simulink model "stateSpaceModel"  (R2025a)
settings: Solver=VariableStepAuto  StartTime=0.0  StopTime=10.0  RelTol=1e-3
PreLoadFcn:
  | run motor_specs.m
values from neighbouring files (symbols this model uses):
  J = 6.3E-6    (= 6.3e-06)    [motor_specs.m]
  L = 0.000238    [motor_specs.m]
  R = 3.23    [motor_specs.m]
undefined symbols (not defined in the file or in its folder): b, k_e, k_m, U_0
settings Model: Creator=aladdin  LastModifiedBy=aladdin

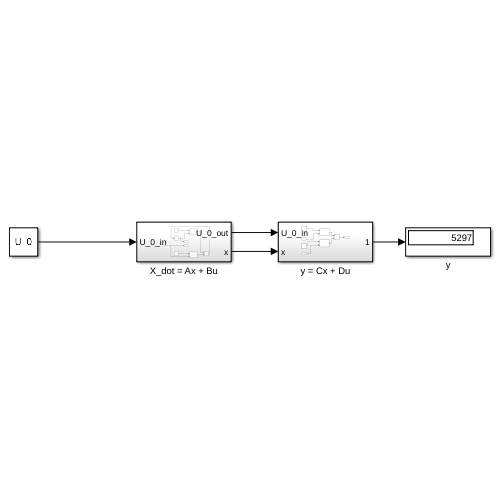
[thumbnail: Simulink's stored preview of the top-level diagram]
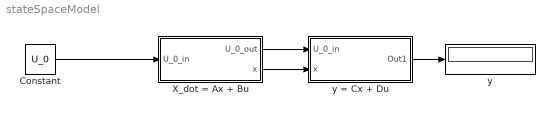
== system stateSpaceModel ==
  Constant : Constant  Value=U_0
  X_dot = Ax + Bu : Subsystem
  y : Display
  y = Cx + Du : Subsystem
  wires:
  Constant/1 -> X_dot = Ax + Bu/1(U_0_in)
  X_dot = Ax + Bu/1(U_0_out) -> y = Cx + Du/1(U_0_in)
  X_dot = Ax + Bu/2(x) -> y = Cx + Du/2(x)
  y = Cx + Du/1(Out1) -> y/1

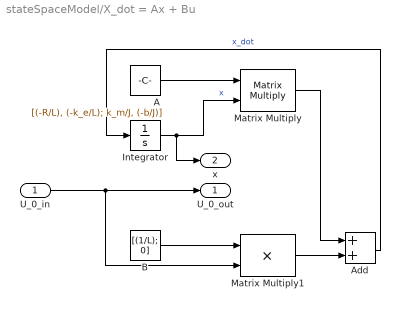
== system stateSpaceModel/X_dot = Ax + Bu ==
  U_0_in : Inport
  A : Constant  Value=[(-R/L), (-k_e/L); k_m/J, (-b/J)]
  Add : Sum
  B : Constant  Value=[(1/L); 0]  VectorParams1D=off
  Integrator : Integrator
  Matrix Multiply : Product  Multiplication=Matrix(*)
  Matrix Multiply1 : Product
  U_0_out : Outport
  x : Outport  Port=2
  wires:
  U_0_in/1 -> Matrix Multiply1/2, U_0_out/1
  A/1 -> Matrix Multiply/1
  Matrix Multiply/1 -> Add/1
  Add/1 -> Integrator/1  "x_dot"
  Integrator/1 -> x/1, Matrix Multiply/2  "x"
  B/1 -> Matrix Multiply1/1
  Matrix Multiply1/1 -> Add/2

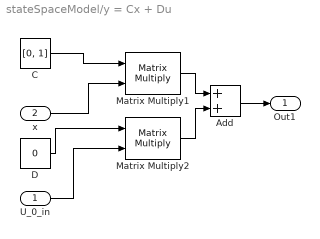
== system stateSpaceModel/y = Cx + Du ==
  U_0_in : Inport
  x : Inport  Port=2
  Add : Sum
  C : Constant  Value=[0, 1]  VectorParams1D=off
  D : Constant  Value=0
  Matrix Multiply1 : Product  Multiplication=Matrix(*)
  Matrix Multiply2 : Product  Multiplication=Matrix(*)
  Out1 : Outport
  wires:
  U_0_in/1 -> Matrix Multiply2/2
  C/1 -> Matrix Multiply1/1
  x/1 -> Matrix Multiply1/2
  Matrix Multiply1/1 -> Add/1
  D/1 -> Matrix Multiply2/1
  Matrix Multiply2/1 -> Add/2
  Add/1 -> Out1/1
